simulink library "pacejka_trans"  (R2020b)
settings: Solver=ode45  StartTime=0.0  StopTime=10.0  RelTol=1e-3  EnableMultiTasking=on
undefined symbols (not defined in the file): DiscIntNeverNeededParam, par_TIR, UC_TireFy
libraries: simulink x2, $bdroot x1
(part 1 of 2)
settings Model: Creator=schultze  LastModifiedBy=ga69qig
settings DataIOCC: LimitDataPoints=on  SaveFormat=Array  SignalLoggingSaveFormat=ModelDataLogs  ReturnWorkspaceOutputs=off
settings OptimizationCC: ExpressionDepthLimit=2147483647  LifeSpan=inf
settings DebuggingCC: UnderspecifiedInitializationDetection=Classic  MergeDetectMultiDrivingBlocksExec=none  SolverPrmCheckMsg=warning  FcnCallInpInsideContextMsg=warning  AllowSymbolicDim=off  StateNameClashWarn=warning  SFUnexpectedBacktrackingDiag=warning  SFNoUnconditionalDefaultTransitionDiag=warning  SFExecutionAtInitializationDiag=none  ArithmeticOperatorsInVariantConditions=warning
settings HardwareCC: ProdBitPerPointer=32  ProdBitPerSizeT=32  ProdBitPerPtrDiffT=32  ProdLargestAtomicFloat=None  ProdIntDivRoundTo=Undefined  ProdEndianess=Unspecified  ProdWordSize=32  ProdHWDeviceType=32-bit Generic
settings ModelReferenceCC: PropagateSignalLabelsOutOfModel=off
settings SFSimCC: SimUseLocalCustomCode=off  CustomCodeUndefinedFunction=UseInterfaceOnly
settings RTWCC: RTWUseLocalCustomCode=off
settings CodeAppCC: StateflowObjectComments=on
settings GRTTargetCC: TargetLangStandard=C89/C90 (ANSI)  CombineOutputUpdateFcns=off  GRTInterface=on
settings ConfigComp: CovMetricSettings=dw  CovSaveCumulativeToWorkspaceVar=on  CovSaveSingleToWorkspaceVar=on  CovExternalEMLEnable=off

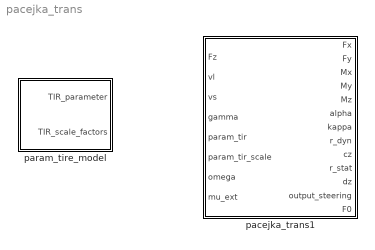
== system pacejka_trans ==
  pacejka_trans1 : Subsystem  mask{mounted_side_input=right}
      mask prompts: mounted_side_input "mounted side"
      mask init:
      | switch mounted_side_input
      |     case 1
      |         mounted_side=0;
      |     case 2
      |         mounted_side=1;
      |     case 3
      |         mounted_side=-1;
      | end
      mask TypeOptions mounted_side_input: undefined | left | right
  param_tire_model : Subsystem

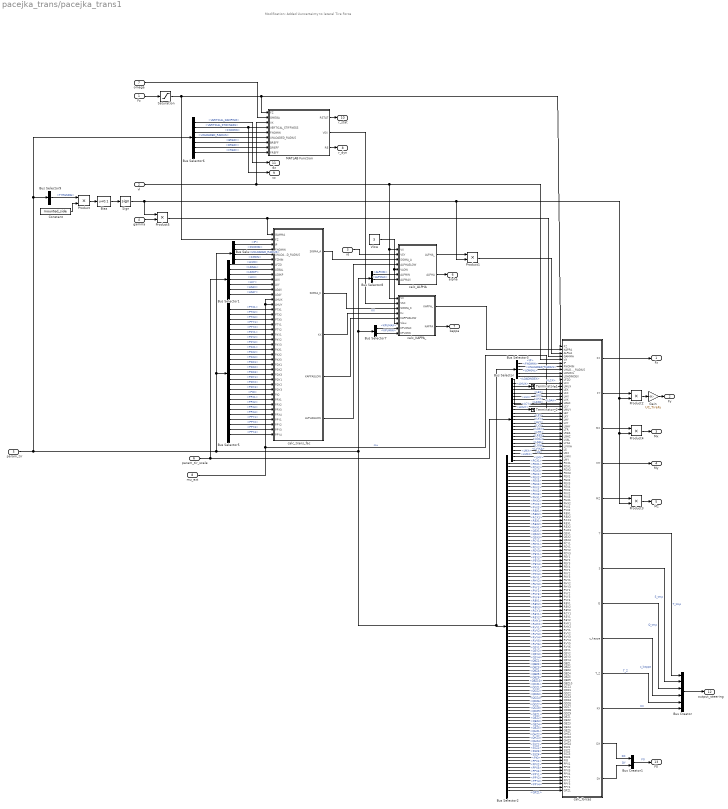
== system pacejka_trans/pacejka_trans1 ==
  note: Modification: Added Uuncertainty to lateral Tire Force
  Fz : Inport
  vl : Inport  Port=2
  vs : Inport  Port=3
  gamma : Inport  Port=4
  param_tir : Inport  Port=5
  param_tir_scale : Inport  Port=6
  omega : Inport  Port=7
  mu_ext : Inport  Port=8
  Bias : Bias  Bias=0.1
  Bus Creator : BusCreator  Inputs=6
  Bus Creator1 : BusCreator  Inputs=2
  Bus Selector : BusSelector  OutputSignals=LFZO,LCX,LMUX,LEX,LKX,LHX,LVX,LGAX,LCY,LMUY,LEY,LKY,LHY,LVY,LGAY,LTR,LRES,LGAZ,LXAL,LYKA,LVYKA,LS,LMX,LVMX,LMY
  Bus Selector1 : BusSelector  OutputSignals=LFZO,LSGAL,LSGKP,LKX,LKY,LGAX,LGAY
  Bus Selector2 : BusSelector  OutputSignals=PCX1,PDX1,PDX2,PDX3,PEX1,PEX2,PEX3,PEX4,PKX1,PKX2,PKX3,PHX1,PHX2,PVX1,PVX2,RBX1,RBX2,RCX1,REX1,REX2,RHX1,QSX1,QSX2,QSX3,PCY1,PDY1,PDY2,PDY3,PEY1,PEY2,PEY3,PEY4,PKY1,PKY2,PKY3,PHY1,PHY2,PHY3,PVY1,PVY2,PVY3,PVY4,RBY1,RBY2,RBY3,RCY1,REY1,REY2,RHY1,RHY2,RVY1,RVY2,RVY3,RVY4,RVY5,RVY6,QSY1,QSY2,QSY3,QSY4,QBZ1,QBZ2,QBZ3,QBZ4,QBZ5,QBZ9,QBZ10,QCZ1,QDZ1,QDZ2,QDZ3,QDZ4,QDZ6,QDZ7,QDZ8,QDZ9,QEZ1,QEZ2,QEZ3,QEZ4,QEZ5,QHZ1,QHZ2,QHZ3,QHZ4,SSZ1,SSZ2,SSZ3,SSZ4,PIO,PPX1,PPX2,PPX3,PPX4,PPY1,PPY2,PPY3,PPY4,QPZ1
  Bus Selector3 : BusSelector  OutputSignals=IP,FNOMIN,UNLOADED_RADIUS,LONGVL,LOADINDEX
  Bus Selector4 : BusSelector  OutputSignals=IP,FNOMIN,UNLOADED_RADIUS,FZMIN
  Bus Selector5 : BusSelector  OutputSignals=PTX1,PTX2,PTX3,PTY1,PTY2,PKY1,PKY2,PKY3,PKX1,PKX2,PKX3,PDX1,PDX2,PDX3,PDY1,PDY2,PDY3,PIO,PPX1,PPX2,PPX3,PPX4,PPY1,PPY2,PPY3,PPY4
  Bus Selector6 : BusSelector  OutputSignals=VERTICAL_DAMPING,VERTICAL_STIFFNESS,FNOMIN,UNLOADED_RADIUS,BREFF,DREFF,FREFF
  Bus Selector7 : BusSelector  OutputSignals=KPUMAX,KPUMIN
  Bus Selector8 : BusSelector  OutputSignals=ALPMIN,ALPMAX
  Bus Selector9 : BusSelector  OutputSignals=TYRESIDE
  Constant : Constant  Value=mounted_side
  Gain : Gain  Gain=UC_TireFy
  MATLAB Function : MATLAB Function  TreatAsAtomicUnit=on
  Product{,1..5} (6 alike) : Product  RndMeth=Zero
  Saturation : Saturate  UpperLimit=99999999  LowerLimit=0.001
  Sign : Signum
  Terminator_1 : Terminator
  Terminator_2 : Terminator
  Vlow : Constant  Value=3
  calc_ALPHA : Subsystem
  calc_KAPPA_ : Subsystem
  calc_forces : MATLAB Function  TreatAsAtomicUnit=on
  calc_trans_fac : MATLAB Function  TreatAsAtomicUnit=on
  Fx : Outport  VectorParamsAs1DForOutWhenUnconnected=off
  Fy : Outport  Port=2  VectorParamsAs1DForOutWhenUnconnected=off
  Mx : Outport  Port=3  VectorParamsAs1DForOutWhenUnconnected=off
  My : Outport  Port=4  VectorParamsAs1DForOutWhenUnconnected=off
  Mz : Outport  Port=5  VectorParamsAs1DForOutWhenUnconnected=off
  alpha : Outport  Port=6  VectorParamsAs1DForOutWhenUnconnected=off
  kappa : Outport  Port=7  VectorParamsAs1DForOutWhenUnconnected=off
  r_dyn : Outport  Port=8  VectorParamsAs1DForOutWhenUnconnected=off
  cz : Outport  Port=9  VectorParamsAs1DForOutWhenUnconnected=off
  r_stat : Outport  Port=10  VectorParamsAs1DForOutWhenUnconnected=off
  dz : Outport  Port=11  VectorParamsAs1DForOutWhenUnconnected=off
  output_steering : Outport  Port=12  VectorParamsAs1DForOutWhenUnconnected=off
  F0 : Outport  Port=13  VectorParamsAs1DForOutWhenUnconnected=off
  wires:
  Bus Creator1/1 -> F0/1  "F0"
  calc_forces/13(DY) -> Bus Creator1/2  "DY"
  calc_forces/12(DX) -> Bus Creator1/1  "DX"
  Bus Selector/25 -> calc_forces/35(LMY)  "<LMY>"
  calc_forces/11(KX) -> Bus Creator/6  "KX"
  Bus Selector4/1 -> calc_trans_fac/3(IP)  "<IP>"
  Bus Selector5/26 -> calc_trans_fac/41(PPY4)  "<PPY4>"
  Bus Selector5/25 -> calc_trans_fac/40(PPY3)  "<PPY3>"
  Bus Selector5/24 -> calc_trans_fac/39(PPY2)  "<PPY2>"
  Bus Selector5/23 -> calc_trans_fac/38(PPY1)  "<PPY1>"
  Bus Selector5/22 -> calc_trans_fac/37(PPX4)  "<PPX4>"
  Bus Selector5/21 -> calc_trans_fac/36(PPX3)  "<PPX3>"
  Bus Selector5/20 -> calc_trans_fac/35(PPX2)  "<PPX2>"
  Bus Selector5/19 -> calc_trans_fac/34(PPX1)  "<PPX1>"
  Bus Selector5/18 -> calc_trans_fac/33(PIO)  "<PIO>"
  Bus Selector3/1 -> calc_forces/6(IP)  "<IP>"
  Bus Selector3/5 -> calc_forces/10(LOADINDEX)  "<LOADINDEX>"
  Bus Selector3/4 -> calc_forces/9(LONGVL)  "<LONGVL>"
  Bus Selector2/99 -> calc_forces/134(QPZ1)  "<QPZ1>"
  Bus Selector2/98 -> calc_forces/133(PPY4)  "<PPY4>"
  Bus Selector2/97 -> calc_forces/132(PPY3)  "<PPY3>"
  Bus Selector2/96 -> calc_forces/131(PPY2)  "<PPY2>"
  Bus Selector2/95 -> calc_forces/130(PPY1)  "<PPY1>"
  Bus Selector2/94 -> calc_forces/129(PPX4)  "<PPX4>"
  Bus Selector2/93 -> calc_forces/128(PPX3)  "<PPX3>"
  Bus Selector2/92 -> calc_forces/127(PPX2)  "<PPX2>"
  Bus Selector2/91 -> calc_forces/126(PPX1)  "<PPX1>"
  Bus Selector2/90 -> calc_forces/125(PIO)  "<PIO>"
  calc_forces/10(T_Z) -> Bus Creator/5  "T_Z"
  calc_forces/9(c_kappa) -> Bus Creator/4  "c_kappa"
  Bus Creator/1 -> output_steering/1
  gamma/1 -> Product5/2
  calc_KAPPA_/2(KAPPA) -> kappa/1
  mu_ext/1 -> calc_forces/13(LMUX), calc_forces/20(LMUY), calc_trans_fac/15(LMUY), calc_trans_fac/14(LMUX)  "mu"
  Vlow/1 -> calc_ALPHA/5(VLOW), calc_KAPPA_/6(Vlow)
  Bus Selector1/5 -> calc_trans_fac/11(LKY)  "<LKY>"
  calc_trans_fac/5(ALPHASLOW) -> calc_ALPHA/4(ALPHASLOW)
  Bus Selector5/7 -> calc_trans_fac/22(PKY2)  "<PKY2>"
  Bus Selector5/6 -> calc_trans_fac/21(PKY1)  "<PKY1>"
  Bus Selector5/17 -> calc_trans_fac/32(PDY3)  "<PDY3>"
  Bus Selector5/16 -> calc_trans_fac/31(PDY2)  "<PDY2>"
  Bus Selector5/15 -> calc_trans_fac/30(PDY1)  "<PDY1>"
  Bus Selector1/7 -> calc_trans_fac/13(LGAY)  "<LGAY>"
  calc_trans_fac/4(KAPPASLOW) -> calc_KAPPA_/5(KAPPASLOW)
  Bus Selector5/14 -> calc_trans_fac/29(PDX3)  "<PDX3>"
  Bus Selector5/13 -> calc_trans_fac/28(PDX2)  "<PDX2>"
  Bus Selector5/12 -> calc_trans_fac/27(PDX1)  "<PDX1>"
  Bus Selector1/6 -> calc_trans_fac/12(LGAX)  "<LGAX>"
  Bus Selector5/11 -> calc_trans_fac/26(PKX3)  "<PKX3>"
  Bus Selector5/10 -> calc_trans_fac/25(PKX2)  "<PKX2>"
  Bus Selector5/9 -> calc_trans_fac/24(PKX1)  "<PKX1>"
  Bus Selector1/4 -> calc_trans_fac/10(LKX)  "<LKX>"
  calc_trans_fac/3(KX) -> calc_KAPPA_/4(Kx)  "KX"
  vl/1 -> calc_forces/5(VX), calc_ALPHA/1(VX), calc_KAPPA_/1(VX), MATLAB Function/3(VX)
  Bus Selector6/7 -> MATLAB Function/9(FREFF)  "<FREFF>"
  Bus Selector6/6 -> MATLAB Function/8(DREFF)  "<DREFF>"
  Bus Selector6/5 -> MATLAB Function/7(BREFF)  "<BREFF>"
  Bus Selector4/4 -> calc_trans_fac/6(FZMIN)  "<FZMIN>"
  calc_ALPHA/1(ALPHA_) -> Product1/1
  calc_trans_fac/1(SIGMA_A) -> calc_ALPHA/3(SIGMA_A)
  calc_trans_fac/2(SIGMA_K) -> calc_KAPPA_/3(SIGMA_K)
  vs/1 -> calc_ALPHA/2(VSY)
  Fz/1 -> Saturation/1
  Product5/1 -> calc_forces/4(GAMMA), calc_trans_fac/1(GAMMA)
  param_tir_scale/1 -> Bus Selector/1, Bus Selector1/1
  Bus Selector/1 -> calc_forces/11(LFZO)  "<LFZO>"
  Bus Selector/2 -> calc_forces/12(LCX)  "<LCX>"
  Bus Selector/4 -> calc_forces/14(LEX)  "<LEX>"
  Bus Selector/5 -> calc_forces/15(LKX)  "<LKX>"
  Bus Selector/6 -> calc_forces/16(LHX)  "<LHX>"
  Bus Selector/7 -> calc_forces/17(LVX)  "<LVX>"
  Bus Selector/8 -> calc_forces/18(LGAX)  "<LGAX>"
  Bus Selector/9 -> calc_forces/19(LCY)  "<LCY>"
  Bus Selector/11 -> calc_forces/21(LEY)  "<LEY>"
  Bus Selector/12 -> calc_forces/22(LKY)  "<LKY>"
  Bus Selector/13 -> calc_forces/23(LHY)  "<LHY>"
  Bus Selector/14 -> calc_forces/24(LVY)  "<LVY>"
  Bus Selector/15 -> calc_forces/25(LGAY)  "<LGAY>"
  Bus Selector/16 -> calc_forces/26(LTR)  "<LTR>"
  Bus Selector/17 -> calc_forces/27(LRES)  "<LRES>"
  Bus Selector/18 -> calc_forces/28(LGAZ)  "<LGAZ>"
  Bus Selector/19 -> calc_forces/29(LXAL)  "<LXAL>"
  Bus Selector/20 -> calc_forces/30(LYKA)  "<LYKA>"
  Bus Selector/21 -> calc_forces/31(LVYKA)  "<LVYKA>"
  Bus Selector/22 -> calc_forces/32(LS)  "<LS>"
  Bus Selector/23 -> calc_forces/33(LMX)  "<LMX>"
  Bus Selector/24 -> calc_forces/34(LVMX)  "<LVMX>"
  Bus Selector1/1 -> calc_trans_fac/7(LFZO)  "<LFZO>"
  Bus Selector1/2 -> calc_trans_fac/8(LSGAL)  "<LSGAL>"
  Bus Selector1/3 -> calc_trans_fac/9(LSGKP)  "<LSGKP>"
  param_tir/1 -> Bus Selector2/1, Bus Selector3/1, Bus Selector7/1, Bus Selector8/1, Bus Selector5/1, Bus Selector4/1, Bus Selector6/1, Bus Selector9/1
  Bus Selector3/2 -> calc_forces/7(FNOMIN)  "<FNOMIN>"
  Bus Selector3/3 -> calc_forces/8(UNLOADED_RADIUS)  "<UNLOADED_RADIUS>"
  Bus Selector2/1 -> calc_forces/36(PCX1)  "<PCX1>"
  Bus Selector2/2 -> calc_forces/37(PDX1)  "<PDX1>"
  Bus Selector2/3 -> calc_forces/38(PDX2)  "<PDX2>"
  Bus Selector2/4 -> calc_forces/39(PDX3)  "<PDX3>"
  Bus Selector2/5 -> calc_forces/40(PEX1)  "<PEX1>"
  Bus Selector2/6 -> calc_forces/41(PEX2)  "<PEX2>"
  Bus Selector2/7 -> calc_forces/42(PEX3)  "<PEX3>"
  Bus Selector2/8 -> calc_forces/43(PEX4)  "<PEX4>"
  Bus Selector2/9 -> calc_forces/44(PKX1)  "<PKX1>"
  Bus Selector2/10 -> calc_forces/45(PKX2)  "<PKX2>"
  Bus Selector2/11 -> calc_forces/46(PKX3)  "<PKX3>"
  Bus Selector2/12 -> calc_forces/47(PHX1)  "<PHX1>"
  Bus Selector2/13 -> calc_forces/48(PHX2)  "<PHX2>"
  Bus Selector2/14 -> calc_forces/49(PVX1)  "<PVX1>"
  Bus Selector2/15 -> calc_forces/50(PVX2)  "<PVX2>"
  Bus Selector2/16 -> calc_forces/51(RBX1)  "<RBX1>"
  Bus Selector2/17 -> calc_forces/52(RBX2)  "<RBX2>"
  Bus Selector2/18 -> calc_forces/53(RCX1)  "<RCX1>"
  Bus Selector2/19 -> calc_forces/54(REX1)  "<REX1>"
  Bus Selector2/20 -> calc_forces/55(REX2)  "<REX2>"
  Bus Selector2/21 -> calc_forces/56(RHX1)  "<RHX1>"
  Bus Selector2/22 -> calc_forces/57(QSX1)  "<QSX1>"
  Bus Selector2/23 -> calc_forces/58(QSX2)  "<QSX2>"
  Bus Selector2/24 -> calc_forces/59(QSX3)  "<QSX3>"
  Bus Selector2/25 -> calc_forces/60(PCY1)  "<PCY1>"
  Bus Selector2/26 -> calc_forces/61(PDY1)  "<PDY1>"
  Bus Selector2/27 -> calc_forces/62(PDY2)  "<PDY2>"
  Bus Selector2/28 -> calc_forces/63(PDY3)  "<PDY3>"
  Bus Selector2/29 -> calc_forces/64(PEY1)  "<PEY1>"
  Bus Selector2/30 -> calc_forces/65(PEY2)  "<PEY2>"
  Bus Selector2/31 -> calc_forces/66(PEY3)  "<PEY3>"
  Bus Selector2/32 -> calc_forces/67(PEY4)  "<PEY4>"
  Bus Selector2/33 -> calc_forces/68(PKY1)  "<PKY1>"
  Bus Selector2/34 -> calc_forces/69(PKY2)  "<PKY2>"
  Bus Selector2/35 -> calc_forces/70(PKY3)  "<PKY3>"
  Bus Selector2/36 -> calc_forces/71(PHY1)  "<PHY1>"
  Bus Selector2/37 -> calc_forces/72(PHY2)  "<PHY2>"
  Bus Selector2/38 -> calc_forces/73(PHY3)  "<PHY3>"
  Bus Selector2/39 -> calc_forces/74(PVY1)  "<PVY1>"
  Bus Selector2/40 -> calc_forces/75(PVY2)  "<PVY2>"
  Bus Selector2/41 -> calc_forces/76(PVY3)  "<PVY3>"
  Bus Selector2/42 -> calc_forces/77(PVY4)  "<PVY4>"
  Bus Selector2/43 -> calc_forces/78(RBY1)  "<RBY1>"
  Bus Selector2/44 -> calc_forces/79(RBY2)  "<RBY2>"
  Bus Selector2/45 -> calc_forces/80(RBY3)  "<RBY3>"
  Bus Selector2/46 -> calc_forces/81(RCY1)  "<RCY1>"
  Bus Selector2/47 -> calc_forces/82(REY1)  "<REY1>"
  Bus Selector2/48 -> calc_forces/83(REY2)  "<REY2>"
  Bus Selector2/49 -> calc_forces/84(RHY1)  "<RHY1>"
  Bus Selector2/50 -> calc_forces/85(RHY2)  "<RHY2>"
  Bus Selector2/51 -> calc_forces/86(RVY1)  "<RVY1>"
  Bus Selector2/52 -> calc_forces/87(RVY2)  "<RVY2>"
  Bus Selector2/53 -> calc_forces/88(RVY3)  "<RVY3>"
  Bus Selector2/54 -> calc_forces/89(RVY4)  "<RVY4>"
  Bus Selector2/55 -> calc_forces/90(RVY5)  "<RVY5>"
  Bus Selector2/56 -> calc_forces/91(RVY6)  "<RVY6>"
  Bus Selector2/57 -> calc_forces/92(QSY1)  "<QSY1>"
  Bus Selector2/58 -> calc_forces/93(QSY2)  "<QSY2>"
  Bus Selector2/59 -> calc_forces/94(QSY3)  "<QSY3>"
  Bus Selector2/60 -> calc_forces/95(QSY4)  "<QSY4>"
  Bus Selector2/61 -> calc_forces/96(QBZ1)  "<QBZ1>"
  Bus Selector2/62 -> calc_forces/97(QBZ2)  "<QBZ2>"
  Bus Selector2/63 -> calc_forces/98(QBZ3)  "<QBZ3>"
  Bus Selector2/64 -> calc_forces/99(QBZ4)  "<QBZ4>"
  Bus Selector2/65 -> calc_forces/100(QBZ5)  "<QBZ5>"
  Bus Selector2/66 -> calc_forces/101(QBZ9)  "<QBZ9>"
  Bus Selector2/67 -> calc_forces/102(QBZ10)  "<QBZ10>"
  Bus Selector2/68 -> calc_forces/103(QCZ1)  "<QCZ1>"
  Bus Selector2/69 -> calc_forces/104(QDZ1)  "<QDZ1>"
  Bus Selector2/70 -> calc_forces/105(QDZ2)  "<QDZ2>"
  Bus Selector2/71 -> calc_forces/106(QDZ3)  "<QDZ3>"
  Bus Selector2/72 -> calc_forces/107(QDZ4)  "<QDZ4>"
  Bus Selector2/73 -> calc_forces/108(QDZ6)  "<QDZ6>"
  Bus Selector2/74 -> calc_forces/109(QDZ7)  "<QDZ7>"
  Bus Selector2/75 -> calc_forces/110(QDZ8)  "<QDZ8>"
  Bus Selector2/76 -> calc_forces/111(QDZ9)  "<QDZ9>"
  Bus Selector2/77 -> calc_forces/112(QEZ1)  "<QEZ1>"
  Bus Selector2/78 -> calc_forces/113(QEZ2)  "<QEZ2>"
  Bus Selector2/79 -> calc_forces/114(QEZ3)  "<QEZ3>"
  Bus Selector2/80 -> calc_forces/115(QEZ4)  "<QEZ4>"
  Bus Selector2/81 -> calc_forces/116(QEZ5)  "<QEZ5>"
  Bus Selector2/82 -> calc_forces/117(QHZ1)  "<QHZ1>"
  Bus Selector2/83 -> calc_forces/118(QHZ2)  "<QHZ2>"
  Bus Selector2/84 -> calc_forces/119(QHZ3)  "<QHZ3>"
  Bus Selector2/85 -> calc_forces/120(QHZ4)  "<QHZ4>"
  Bus Selector2/86 -> calc_forces/121(SSZ1)  "<SSZ1>"
  Bus Selector2/87 -> calc_forces/122(SSZ2)  "<SSZ2>"
  Bus Selector2/88 -> calc_forces/123(SSZ3)  "<SSZ3>"
  Bus Selector2/89 -> calc_forces/124(SSZ4)  "<SSZ4>"
  Bus Selector5/1 -> calc_trans_fac/16(PTX1)  "<PTX1>"
  Bus Selector5/2 -> calc_trans_fac/17(PTX2)  "<PTX2>"
  Bus Selector5/3 -> calc_trans_fac/18(PTX3)  "<PTX3>"
  Bus Selector5/4 -> calc_trans_fac/19(PTY1)  "<PTY1>"
  Bus Selector5/5 -> calc_trans_fac/20(PTY2)  "<PTY2>"
  Bus Selector5/8 -> calc_trans_fac/23(PKY3)  "<PKY3>"
  Bus Selector4/2 -> calc_trans_fac/4(FNOMIN)  "<FNOMIN>"
  Bus Selector4/3 -> calc_trans_fac/5(UNLOADED_RADIUS)  "<UNLOADED_RADIUS>"
  MATLAB Function/2(VSX) -> calc_KAPPA_/2(VSX)
  Bus Selector6/2 -> MATLAB Function/4(VERTICAL_STIFFNESS), cz/1  "<VERTICAL_STIFFNESS>"
  Bus Selector6/3 -> MATLAB Function/5(FNOMIN)  "<FNOMIN>"
  Bus Selector6/4 -> MATLAB Function/6(UNLOADED_RADIUS)  "<UNLOADED_RADIUS>"
  omega/1 -> MATLAB Function/2(OMEGA)
  MATLAB Function/3(RE) -> r_dyn/1
  calc_forces/4(MY) -> My/1
  calc_forces/1(FX) -> Fx/1
  Bus Selector/10 -> Terminator_2/1  "<LMUY>"
  Bus Selector7/1 -> calc_KAPPA_/7(KPUMAX)  "<KPUMAX>"
  Bus Selector7/2 -> calc_KAPPA_/8(KPUMIN)  "<KPUMIN>"
  Bus Selector8/1 -> calc_ALPHA/6(ALPMIN)  "<ALPMIN>"
  Bus Selector8/2 -> calc_ALPHA/7(ALPMAX)  "<ALPMAX>"
  Product1/1 -> calc_forces/3(ALPHA)
  Bus Selector/3 -> Terminator_1/1  "<LMUX>"
  Bus Selector9/1 -> Product/1  "<TYRESIDE>"
  Constant/1 -> Product/2
  Product/1 -> Bias/1
  Bias/1 -> Sign/1
  Sign/1 -> Product1/2, Product3/2, Product4/2, Product2/2, Product5/1
  Product2/1 -> Gain/1
  Product3/1 -> Mz/1
  calc_forces/5(MZ) -> Product3/1
  Product4/1 -> Mx/1
  calc_forces/3(MX) -> Product4/1
  MATLAB Function/1(RSTAT) -> r_stat/1
  Bus Selector6/1 -> dz/1  "<VERTICAL_DAMPING>"
  Saturation/1 -> calc_forces/1(FZ), MATLAB Function/1(FZ), calc_trans_fac/2(FZ)
  calc_forces/2(FY) -> Product2/1
  calc_ALPHA/2(ALPHA) -> alpha/1
  calc_forces/6(T) -> Bus Creator/1  "T_tmp"
  calc_forces/7(S) -> Bus Creator/2  "S_tmp"
  calc_forces/8(Q) -> Bus Creator/3  "Q_tmp"
  calc_KAPPA_/1(KAPPA_) -> calc_forces/2(KAPPA)
  Gain/1 -> Fy/1

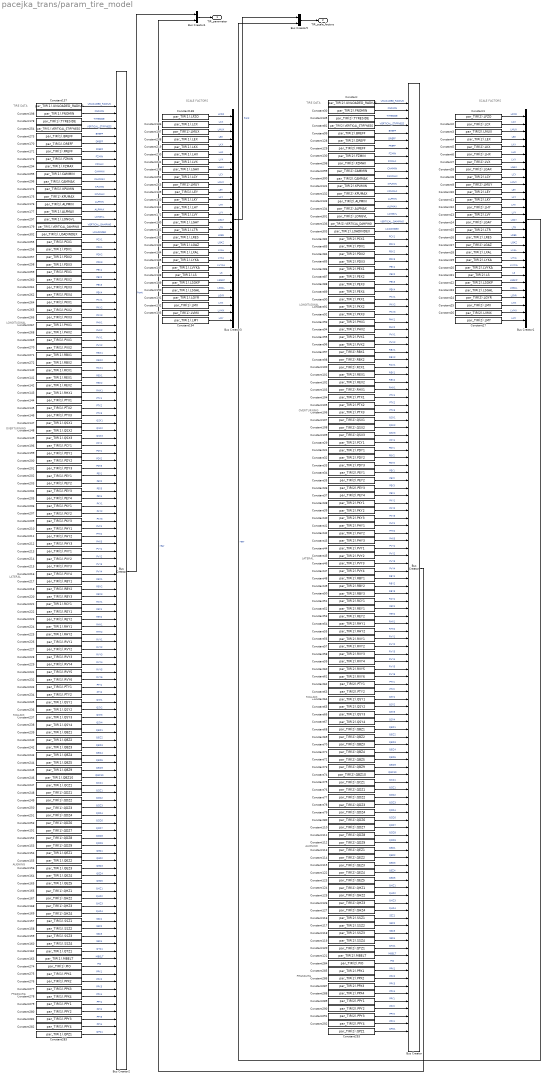
== system pacejka_trans/param_tire_model ==
  note: SCALE FACTORS
  note: TIRE DATA
  note: LONGITUDINAL
  note: LATERAL
  note: OVERTURNING
  note: ROLLING
  note: ALIGNING
  note: SCALE FACTORS
  note: TIRE DATA
  note: LONGITUDINAL
  note: LATERAL
  note: OVERTURNING
  note: ROLLING
  note: ALIGNING
  note: PRESSURE
  note: PRESSURE
  Bus Creator : BusCreator  Inputs=124
  Bus Creator1 : BusCreator  Inputs=28
  Bus Creator2 : BusCreator  Inputs=124
  Bus Creator3 : BusCreator  Inputs=28
  Bus Creator4 : BusCreator  Inputs=2
  Bus Creator5 : BusCreator  Inputs=2
  Constant : Constant  Value=par_TIR(2).UNLOADED_RADIUS
  Constant1 : Constant  Value=par_TIR(2).LFZO
  Constant10 : Constant  Value=par_TIR(2).LEY
  Constant100 : Constant  Value=par_TIR(2).RCX1
  Constant101 : Constant  Value=par_TIR(2).REX1
  Constant102 : Constant  Value=par_TIR(2).REX2
  Constant103 : Constant  Value=par_TIR(2).RHX1
  Constant104 : Constant  Value=par_TIR(2).PTX1
  Constant105 : Constant  Value=par_TIR(2).PTX2
  Constant106 : Constant  Value=par_TIR(2).PTX3
  Constant107 : Constant  Value=par_TIR(2).QSX1
  Constant108 : Constant  Value=par_TIR(2).QSX2
  Constant109 : Constant  Value=par_TIR(2).QSX3
  Constant11 : Constant  Value=par_TIR(2).LKY
  Constant110 : Constant  Value=par_TIR(2).QDZ7
  Constant111 : Constant  Value=par_TIR(2).QDZ8
  Constant112 : Constant  Value=par_TIR(2).QDZ9
  Constant113 : Constant  Value=par_TIR(2).QEZ1
  Constant114 : Constant  Value=par_TIR(2).QEZ2
  Constant115 : Constant  Value=par_TIR(2).QEZ3
  Constant116 : Constant  Value=par_TIR(2).SSZ1
  Constant117 : Constant  Value=par_TIR(2).SSZ2
  Constant118 : Constant  Value=par_TIR(2).SSZ3
  Constant119 : Constant  Value=par_TIR(2).SSZ4
  Constant12 : Constant  Value=par_TIR(2).LHY
  Constant120 : Constant  Value=par_TIR(2).QTZ1
  Constant121 : Constant  Value=par_TIR(2).MBELT
  Constant122 : Constant  Value=par_TIR(2).QEZ4
  Constant123 : Constant  Value=par_TIR(2).QEZ5
  Constant124 : Constant  Value=par_TIR(2).QHZ1
  Constant125 : Constant  Value=par_TIR(2).QHZ2
  Constant126 : Constant  Value=par_TIR(2).QHZ3
  Constant127 : Constant  Value=par_TIR(2).QHZ4
  Constant128 : Constant  Value=par_TIR(2).DREFF
  Constant129 : Constant  Value=par_TIR(2).FREFF
  Constant13 : Constant  Value=par_TIR(2).LVY
  Constant130 : Constant  Value=par_TIR(2).FZMIN
  Constant131 : Constant  Value=par_TIR(2).KPUMIN
  Constant132 : Constant  Value=par_TIR(2).KPUMAX
  Constant133 : Constant  Value=par_TIR(2).ALPMIN
  Constant134 : Constant  Value=par_TIR(2).ALPMAX
  Constant135 : Constant  Value=par_TIR(2).TYRESIDE
  Constant136 : Constant  Value=par_TIR(2).VERTICAL_DAMPING
  Constant137 : Constant  Value=par_TIR(1).UNLOADED_RADIUS
  Constant138 : Constant  Value=par_TIR(1).LFZO
  Constant139 : Constant  Value=par_TIR(1).LEY
  Constant14 : Constant  Value=par_TIR(2).LGAY
  Constant140 : Constant  Value=par_TIR(1).RCX1
  Constant141 : Constant  Value=par_TIR(1).REX1
  Constant142 : Constant  Value=par_TIR(1).REX2
  Constant143 : Constant  Value=par_TIR(1).RHX1
  Constant144 : Constant  Value=par_TIR(1).PTX1
  Constant145 : Constant  Value=par_TIR(1).PTX2
  Constant146 : Constant  Value=par_TIR(1).PTX3
  Constant147 : Constant  Value=par_TIR(1).QSX1
  Constant148 : Constant  Value=par_TIR(1).QSX2
  Constant149 : Constant  Value=par_TIR(1).QSX3
  Constant15 : Constant  Value=par_TIR(2).LTR
  Constant150 : Constant  Value=par_TIR(1).LKY
  Constant151 : Constant  Value=par_TIR(1).QDZ7
  Constant152 : Constant  Value=par_TIR(1).QDZ8
  Constant153 : Constant  Value=par_TIR(1).QDZ9
  Constant154 : Constant  Value=par_TIR(1).QEZ1
  Constant155 : Constant  Value=par_TIR(1).QEZ2
  Constant156 : Constant  Value=par_TIR(1).QEZ3
  Constant157 : Constant  Value=par_TIR(1).SSZ1
  Constant158 : Constant  Value=par_TIR(1).SSZ2
  Constant159 : Constant  Value=par_TIR(1).SSZ3
  Constant16 : Constant  Value=par_TIR(2).LRES
  Constant160 : Constant  Value=par_TIR(1).SSZ4
  Constant161 : Constant  Value=par_TIR(1).LHY
  Constant162 : Constant  Value=par_TIR(1).QTZ1
  Constant163 : Constant  Value=par_TIR(1).MBELT
  Constant164 : Constant  Value=par_TIR(1).QEZ4
  Constant165 : Constant  Value=par_TIR(1).QEZ5
  Constant166 : Constant  Value=par_TIR(1).QHZ1
  Constant167 : Constant  Value=par_TIR(1).QHZ2
  Constant168 : Constant  Value=par_TIR(1).QHZ3
  Constant169 : Constant  Value=par_TIR(1).QHZ4
  Constant17 : Constant  Value=par_TIR(2).LGAZ
  Constant170 : Constant  Value=par_TIR(1).DREFF
  Constant171 : Constant  Value=par_TIR(1).FREFF
  Constant172 : Constant  Value=par_TIR(1).LVY
  Constant173 : Constant  Value=par_TIR(1).FZMIN
  Constant174 : Constant  Value=par_TIR(1).KPUMIN
  Constant175 : Constant  Value=par_TIR(1).KPUMAX
  Constant176 : Constant  Value=par_TIR(1).ALPMIN
  Constant177 : Constant  Value=par_TIR(1).ALPMAX
  Constant178 : Constant  Value=par_TIR(1).TYRESIDE
  Constant179 : Constant  Value=par_TIR(1).VERTICAL_DAMPING
  Constant18 : Constant  Value=par_TIR(2).LXAL
  Constant180 : Constant  Value=par_TIR(1).LGAY
  Constant181 : Constant  Value=par_TIR(1).LTR
  Constant182 : Constant  Value=par_TIR(1).LRES
  Constant183 : Constant  Value=par_TIR(1).LGAZ
  Constant184 : Constant  Value=par_TIR(1).LXAL
  Constant185 : Constant  Value=par_TIR(1).LYKA
  Constant186 : Constant  Value=par_TIR(1).LCX
  Constant187 : Constant  Value=par_TIR(1).LVYKA
  Constant188 : Constant  Value=par_TIR(1).LS
  Constant189 : Constant  Value=par_TIR(1).LSGKP
  Constant19 : Constant  Value=par_TIR(2).LYKA
  Constant190 : Constant  Value=par_TIR(1).LSGAL
  Constant191 : Constant  Value=par_TIR(1).LGYR
  Constant192 : Constant  Value=par_TIR(1).LMX
  Constant193 : Constant  Value=par_TIR(1).LVMX
  Constant194 : Constant  Value=par_TIR(1).LMY
  Constant195 : Constant  Value=par_TIR(1).LGAX
  Constant196 : Constant  Value=par_TIR(1).PCY1
  Constant197 : Constant  Value=par_TIR(1).LMUX
  Constant198 : Constant  Value=par_TIR(1).FNOMIN
  Constant199 : Constant  Value=par_TIR(1).PDY1
  Constant2 : Constant  Value=par_TIR(2).LCX
  Constant20 : Constant  Value=par_TIR(2).LVYKA
  Constant200 : Constant  Value=par_TIR(1).PDY2
  Constant201 : Constant  Value=par_TIR(1).PDY3
  Constant202 : Constant  Value=par_TIR(1).PEY1
  Constant203 : Constant  Value=par_TIR(1).PEY2
  Constant204 : Constant  Value=par_TIR(1).PEY3
  Constant205 : Constant  Value=par_TIR(1).PEY4
  Constant206 : Constant  Value=par_TIR(1).PKY1
  Constant207 : Constant  Value=par_TIR(1).PKY2
  Constant208 : Constant  Value=par_TIR(1).LEX
  Constant209 : Constant  Value=par_TIR(1).PKY3
  Constant21 : Constant  Value=par_TIR(2).LS
  Constant210 : Constant  Value=par_TIR(1).PHY1
  Constant211 : Constant  Value=par_TIR(1).PHY2
  Constant212 : Constant  Value=par_TIR(1).PHY3
  Constant213 : Constant  Value=par_TIR(1).PVY1
  Constant214 : Constant  Value=par_TIR(1).PVY2
  Constant215 : Constant  Value=par_TIR(1).PVY3
  Constant216 : Constant  Value=par_TIR(1).PVY4
  Constant217 : Constant  Value=par_TIR(1).RBY1
  Constant218 : Constant  Value=par_TIR(1).RBY2
  Constant219 : Constant  Value=par_TIR(1).LKX
  Constant22 : Constant  Value=par_TIR(2).LSGKP
  Constant220 : Constant  Value=par_TIR(1).RBY3
  Constant221 : Constant  Value=par_TIR(1).RCY1
  Constant222 : Constant  Value=par_TIR(1).REY1
  Constant223 : Constant  Value=par_TIR(1).REY2
  Constant224 : Constant  Value=par_TIR(1).RHY1
  Constant225 : Constant  Value=par_TIR(1).RHY2
  Constant226 : Constant  Value=par_TIR(1).RVY1
  Constant227 : Constant  Value=par_TIR(1).RVY2
  Constant228 : Constant  Value=par_TIR(1).RVY3
  Constant229 : Constant  Value=par_TIR(1).RVY4
  Constant23 : Constant  Value=par_TIR(2).LSGAL
  Constant230 : Constant  Value=par_TIR(1).LHX
  Constant231 : Constant  Value=par_TIR(1).RVY5
  Constant232 : Constant  Value=par_TIR(1).RVY6
  Constant233 : Constant  Value=par_TIR(1).PTY1
  Constant234 : Constant  Value=par_TIR(1).PTY2
  Constant235 : Constant  Value=par_TIR(1).QSY1
  Constant236 : Constant  Value=par_TIR(1).QSY2
  Constant237 : Constant  Value=par_TIR(1).QSY3
  Constant238 : Constant  Value=par_TIR(1).QSY4
  Constant239 : Constant  Value=par_TIR(1).QBZ1
  Constant24 : Constant  Value=par_TIR(2).LGYR
  Constant240 : Constant  Value=par_TIR(1).QBZ2
  Constant241 : Constant  Value=par_TIR(1).LVX
  Constant242 : Constant  Value=par_TIR(1).QBZ3
  Constant243 : Constant  Value=par_TIR(1).QBZ4
  Constant244 : Constant  Value=par_TIR(1).QBZ5
  Constant245 : Constant  Value=par_TIR(1).QBZ9
  Constant246 : Constant  Value=par_TIR(1).QBZ10
  Constant247 : Constant  Value=par_TIR(1).QCZ1
  Constant248 : Constant  Value=par_TIR(1).QDZ1
  Constant249 : Constant  Value=par_TIR(1).QDZ2
  Constant25 : Constant  Value=par_TIR(2).LMX
  Constant250 : Constant  Value=par_TIR(1).QDZ3
  Constant251 : Constant  Value=par_TIR(1).QDZ4
  Constant252 : Constant  Value=par_TIR(1).LCY
  Constant253 : Constant  Value=par_TIR(1).QDZ6
  Constant254 : Constant  Value=par_TIR(1).VERTICAL_STIFFNESS
  Constant255 : Constant  Value=par_TIR(1).PCX1
  Constant256 : Constant  Value=par_TIR(1).PDX1
  Constant257 : Constant  Value=par_TIR(1).PDX2
  Constant258 : Constant  Value=par_TIR(1).PDX3
  Constant259 : Constant  Value=par_TIR(1).PEX1
  Constant26 : Constant  Value=par_TIR(2).LVMX
  Constant260 : Constant  Value=par_TIR(1).PEX2
  Constant261 : Constant  Value=par_TIR(1).PEX3
  Constant262 : Constant  Value=par_TIR(1).PEX4
  Constant263 : Constant  Value=par_TIR(1).LMUY
  Constant264 : Constant  Value=par_TIR(1).PKX1
  Constant265 : Constant  Value=par_TIR(1).PKX2
  Constant266 : Constant  Value=par_TIR(1).PKX3
  Constant267 : Constant  Value=par_TIR(1).PHX1
  Constant268 : Constant  Value=par_TIR(1).PHX2
  Constant269 : Constant  Value=par_TIR(1).PVX1
  Constant27 : Constant  Value=par_TIR(2).LMY
  Constant270 : Constant  Value=par_TIR(1).PVX2
  Constant271 : Constant  Value=par_TIR(1).RBX1
  Constant272 : Constant  Value=par_TIR(1).RBX2
  Constant273 : Constant  Value=par_TIR(1).BREFF
  Constant274 : Constant  RequirementInfo="{}  %GIDa_26266586_498b_462f_b489_3d0c6574960f"  Value=par_TIR(1).PIO
  Constant275 : Constant  RequirementInfo={} %GIDa_bd3446b4_e75b_42cc_93fc_63d702bdba05  Value=par_TIR(1).PPX1
  Constant276 : Constant  RequirementInfo={} %GIDa_e7183a53_319d_4b2a_a098_83896b26e061  Value=par_TIR(1).PPX2
  Constant277 : Constant  RequirementInfo={} %GIDa_4d8b6861_cb82_4b47_965b_978958cda42f  Value=par_TIR(1).PPX3
  Constant278 : Constant  RequirementInfo={} %GIDa_c0a2bdc4_fdde_4852_836d_5878f0e5080b  Value=par_TIR(1).PPX4
  Constant279 : Constant  RequirementInfo={} %GIDa_259e4558_aa3a_40ca_8d3a_68c9cc3aff06  Value=par_TIR(1).PPY1
  Constant28 : Constant  Value=par_TIR(2).LGAX
  Constant280 : Constant  RequirementInfo={} %GIDa_19e9e64b_4c09_4622_8f00_2f4be9e7e16b  Value=par_TIR(1).PPY2
  Constant281 : Constant  RequirementInfo={} %GIDa_9a02291b_2d1e_49a5_a1e4_b19d87d3265f  Value=par_TIR(1).PPY3
  Constant282 : Constant  RequirementInfo={} %GIDa_ecd77677_9c33_4f16_bf1f_0a0632ce1b6d  Value=par_TIR(1).PPY4
  Constant283 : Constant  RequirementInfo={} %GIDa_3542e054_4fbb_4233_8b5e_2c203789807f  Value=par_TIR(1).QPZ1
  Constant284 : Constant  RequirementInfo={} %GIDa_a6cea8bb_6b90_497f_8a27_172ddd318988  Value=par_TIR(2).PIO
  Constant285 : Constant  RequirementInfo={} %GIDa_869ee301_e46e_4e3e_98d5_441bb0b60ee2  Value=par_TIR(2).PPX1
  Constant286 : Constant  RequirementInfo={} %GIDa_2fa7aad5_0b6f_4270_a9fc_fef63194a323  Value=par_TIR(2).PPX2
  Constant287 : Constant  RequirementInfo={} %GIDa_7722773f_46a5_4b48_9921_1b7dc0ffce5d  Value=par_TIR(2).PPX3
  Constant288 : Constant  RequirementInfo={} %GIDa_9b3370dd_7ca6_42c6_ae76_155bd0b3f77a  Value=par_TIR(2).PPX4
  Constant289 : Constant  RequirementInfo={} %GIDa_ebf4fb2f_cc6e_4f60_8b6d_1fa2dededda2  Value=par_TIR(2).PPY1
  Constant29 : Constant  Value=par_TIR(2).PCY1
  Constant290 : Constant  RequirementInfo={} %GIDa_46454242_b81e_41e5_9fcb_0940f6cc9231  Value=par_TIR(2).PPY2
  Constant291 : Constant  RequirementInfo={} %GIDa_9261926a_8ebc_4edf_afdf_1d43d1bd8012  Value=par_TIR(2).PPY3
  Constant292 : Constant  RequirementInfo={} %GIDa_37a6ca2e_28ac_4e3d_851e_41ea970db34f  Value=par_TIR(2).PPY4
  Constant293 : Constant  RequirementInfo={} %GIDa_06c45289_4ba3_4f48_9048_3ee6adfd56e1  Value=par_TIR(2).QPZ1
  Constant294 : Constant  Value=par_TIR(1).FZMAX
  Constant295 : Constant  Value=par_TIR(1).CAMMIN
  Constant296 : Constant  Value=par_TIR(1).CAMMAX
  Constant297 : Constant  Value=par_TIR(1).LONGVL
  Constant298 : Constant  Value=par_TIR(2).FZMAX
  Constant299 : Constant  Value=par_TIR(2).CAMMIN
  Constant3 : Constant  Value=par_TIR(2).LMUX
  Constant30 : Constant  Value=par_TIR(2).FNOMIN
  Constant300 : Constant  Value=par_TIR(2).CAMMAX
  Constant301 : Constant  Value=par_TIR(2).LONGVL
  Constant302 : Constant  Value=par_TIR(1).LOADINDEX
  Constant303 : Constant  Value=par_TIR(2).LOADINDEX
  Constant31 : Constant  Value=par_TIR(2).PDY1
  Constant32 : Constant  Value=par_TIR(2).PDY2
  Constant33 : Constant  Value=par_TIR(2).PDY3
  Constant34 : Constant  Value=par_TIR(2).PEY1
  Constant35 : Constant  Value=par_TIR(2).PEY2
  Constant36 : Constant  Value=par_TIR(2).PEY3
  Constant37 : Constant  Value=par_TIR(2).PEY4
  Constant38 : Constant  Value=par_TIR(2).PKY1
  Constant39 : Constant  Value=par_TIR(2).PKY2
  Constant4 : Constant  Value=par_TIR(2).LEX
  Constant40 : Constant  Value=par_TIR(2).PKY3
  Constant41 : Constant  Value=par_TIR(2).PHY1
  Constant42 : Constant  Value=par_TIR(2).PHY2
  Constant43 : Constant  Value=par_TIR(2).PHY3
  Constant44 : Constant  Value=par_TIR(2).PVY1
  Constant45 : Constant  Value=par_TIR(2).PVY2
  Constant46 : Constant  Value=par_TIR(2).PVY3
  Constant47 : Constant  Value=par_TIR(2).PVY4
  Constant48 : Constant  Value=par_TIR(2).RBY1
  Constant49 : Constant  Value=par_TIR(2).RBY2
  Constant5 : Constant  Value=par_TIR(2).LKX
  Constant50 : Constant  Value=par_TIR(2).RBY3
  Constant51 : Constant  Value=par_TIR(2).RCY1
  Constant52 : Constant  Value=par_TIR(2).REY1
  Constant53 : Constant  Value=par_TIR(2).REY2
  Constant54 : Constant  Value=par_TIR(2).RHY1
  Constant55 : Constant  Value=par_TIR(2).RHY2
  Constant56 : Constant  Value=par_TIR(2).RVY1
  Constant57 : Constant  Value=par_TIR(2).RVY2
  Constant58 : Constant  Value=par_TIR(2).RVY3
  Constant59 : Constant  Value=par_TIR(2).RVY4
  Constant6 : Constant  Value=par_TIR(2).LHX
  Constant60 : Constant  Value=par_TIR(2).RVY5
  Constant61 : Constant  Value=par_TIR(2).RVY6
  Constant62 : Constant  Value=par_TIR(2).PTY1
  Constant63 : Constant  Value=par_TIR(2).PTY2
  Constant64 : Constant  Value=par_TIR(2).QSY1
  Constant65 : Constant  Value=par_TIR(2).QSY2
  Constant66 : Constant  Value=par_TIR(2).QSY3
  Constant67 : Constant  Value=par_TIR(2).QSY4
  Constant68 : Constant  Value=par_TIR(2).QBZ1
  Constant69 : Constant  Value=par_TIR(2).QBZ2
  Constant7 : Constant  Value=par_TIR(2).LVX
  Constant70 : Constant  Value=par_TIR(2).QBZ3
  Constant71 : Constant  Value=par_TIR(2).QBZ4
  Constant72 : Constant  Value=par_TIR(2).QBZ5
  Constant73 : Constant  Value=par_TIR(2).QBZ9
  Constant74 : Constant  Value=par_TIR(2).QBZ10
  Constant75 : Constant  Value=par_TIR(2).QCZ1
  Constant76 : Constant  Value=par_TIR(2).QDZ1
  Constant77 : Constant  Value=par_TIR(2).QDZ2
  Constant78 : Constant  Value=par_TIR(2).QDZ3
  Constant79 : Constant  Value=par_TIR(2).QDZ4
  Constant8 : Constant  Value=par_TIR(2).LCY
  Constant80 : Constant  Value=par_TIR(2).QDZ6
  Constant81 : Constant  Value=par_TIR(2).VERTICAL_STIFFNESS
  Constant82 : Constant  Value=par_TIR(2).PCX1
  Constant83 : Constant  Value=par_TIR(2).PDX1
  Constant84 : Constant  Value=par_TIR(2).PDX2
  Constant85 : Constant  Value=par_TIR(2).PDX3
  Constant86 : Constant  Value=par_TIR(2).PEX1
  Constant87 : Constant  Value=par_TIR(2).PEX2
  Constant88 : Constant  Value=par_TIR(2).PEX3
  Constant89 : Constant  Value=par_TIR(2).PEX4
  Constant9 : Constant  Value=par_TIR(2).LMUY
  Constant90 : Constant  Value=par_TIR(2).PKX1
  Constant91 : Constant  Value=par_TIR(2).PKX2
  Constant92 : Constant  Value=par_TIR(2).PKX3
  Constant93 : Constant  Value=par_TIR(2).PHX1
  Constant94 : Constant  Value=par_TIR(2).PHX2
  Constant95 : Constant  Value=par_TIR(2).PVX1
  Constant96 : Constant  Value=par_TIR(2).PVX2
  Constant97 : Constant  Value=par_TIR(2).RBX1
  Constant98 : Constant  Value=par_TIR(2).RBX2
  Constant99 : Constant  Value=par_TIR(2).BREFF
  TIR_parameter : Outport  VectorParamsAs1DForOutWhenUnconnected=off
  TIR_scale_factors : Outport  Port=2  VectorParamsAs1DForOutWhenUnconnected=off
  wires:
  Bus Creator5/1 -> TIR_scale_factors/1
  Bus Creator3/1 -> Bus Creator5/1  "front"
  Bus Creator4/1 -> TIR_parameter/1
  Bus Creator2/1 -> Bus Creator4/1  "front"
  Constant129/1 -> Bus Creator/7  "FREFF"
  Constant128/1 -> Bus Creator/6  "DREFF"
  Constant99/1 -> Bus Creator/5  "BREFF"
  Constant1/1 -> Bus Creator1/1  "LFZO"
  Constant2/1 -> Bus Creator1/2  "LCX"
  Constant3/1 -> Bus Creator1/3  "LMUX"
  Constant4/1 -> Bus Creator1/4  "LEX"
  Constant5/1 -> Bus Creator1/5  "LKX"
  Constant6/1 -> Bus Creator1/6  "LHX"
  Constant7/1 -> Bus Creator1/7  "LVX"
  Constant28/1 -> Bus Creator1/8  "LGAX"
  Constant8/1 -> Bus Creator1/9  "LCY"
  Constant9/1 -> Bus Creator1/10  "LMUY"
  Constant10/1 -> Bus Creator1/11  "LEY"
  Constant11/1 -> Bus Creator1/12  "LKY"
  Constant12/1 -> Bus Creator1/13  "LHY"
  Constant13/1 -> Bus Creator1/14  "LVY"
  Constant14/1 -> Bus Creator1/15  "LGAY"
  Constant15/1 -> Bus Creator1/16  "LTR"
  Constant16/1 -> Bus Creator1/17  "LRES"
  Constant17/1 -> Bus Creator1/18  "LGAZ"
  Constant18/1 -> Bus Creator1/19  "LXAL"
  Constant19/1 -> Bus Creator1/20  "LYKA"
  Constant20/1 -> Bus Creator1/21  "LVYKA"
  Constant21/1 -> Bus Creator1/22  "LS"
  Constant22/1 -> Bus Creator1/23  "LSGKP"
  Constant23/1 -> Bus Creator1/24  "LSGAL"
  Constant24/1 -> Bus Creator1/25  "LGYR"
  Constant25/1 -> Bus Creator1/26  "LMX"
  Constant26/1 -> Bus Creator1/27  "LVMX"
  Constant27/1 -> Bus Creator1/28  "LMY"
  Bus Creator1/1 -> Bus Creator5/2  "rear"
  Bus Creator/1 -> Bus Creator4/2  "rear"
  Constant/1 -> Bus Creator/1  "UNLOADED_RADIUS"
  Constant30/1 -> Bus Creator/2  "FNOMIN"
  Constant82/1 -> Bus Creator/19  "PCX1"
  Constant83/1 -> Bus Creator/20  "PDX1"
  Constant84/1 -> Bus Creator/21  "PDX2"
  Constant85/1 -> Bus Creator/22  "PDX3"
  Constant86/1 -> Bus Creator/23  "PEX1"
  Constant87/1 -> Bus Creator/24  "PEX2"
  Constant88/1 -> Bus Creator/25  "PEX3"
  Constant89/1 -> Bus Creator/26  "PEX4"
  Constant90/1 -> Bus Creator/27  "PKX1"
  Constant91/1 -> Bus Creator/28  "PKX2"
  Constant92/1 -> Bus Creator/29  "PKX3"
  Constant93/1 -> Bus Creator/30  "PHX1"
  Constant94/1 -> Bus Creator/31  "PHX2"
  Constant95/1 -> Bus Creator/32  "PVX1"
  Constant96/1 -> Bus Creator/33  "PVX2"
  Constant97/1 -> Bus Creator/34  "RBX1"
  Constant98/1 -> Bus Creator/35  "RBX2"
  Constant100/1 -> Bus Creator/36  "RCX1"
  Constant101/1 -> Bus Creator/37  "REX1"
  Constant102/1 -> Bus Creator/38  "REX2"
  Constant103/1 -> Bus Creator/39  "RHX1"
  Constant104/1 -> Bus Creator/40  "PTX1"
  Constant105/1 -> Bus Creator/41  "PTX2"
  Constant106/1 -> Bus Creator/42  "PTX3"
  Constant107/1 -> Bus Creator/43  "QSX1"
  Constant108/1 -> Bus Creator/44  "QSX2"
  Constant109/1 -> Bus Creator/45  "QSX3"
  Constant29/1 -> Bus Creator/46  "PCY1"
  Constant31/1 -> Bus Creator/47  "PDY1"
  Constant32/1 -> Bus Creator/48  "PDY2"
  Constant33/1 -> Bus Creator/49  "PDY3"
  Constant34/1 -> Bus Creator/50  "PEY1"
  Constant35/1 -> Bus Creator/51  "PEY2"
  Constant36/1 -> Bus Creator/52  "PEY3"
  Constant37/1 -> Bus Creator/53  "PEY4"
  Constant38/1 -> Bus Creator/54  "PKY1"
  Constant39/1 -> Bus Creator/55  "PKY2"
  Constant40/1 -> Bus Creator/56  "PKY3"
  Constant41/1 -> Bus Creator/57  "PHY1"
  Constant42/1 -> Bus Creator/58  "PHY2"
  Constant43/1 -> Bus Creator/59  "PHY3"
  Constant44/1 -> Bus Creator/60  "PVY1"
  Constant45/1 -> Bus Creator/61  "PVY2"
  Constant46/1 -> Bus Creator/62  "PVY3"
  Constant47/1 -> Bus Creator/63  "PVY4"
  Constant48/1 -> Bus Creator/64  "RBY1"
  Constant49/1 -> Bus Creator/65  "RBY2"
  Constant50/1 -> Bus Creator/66  "RBY3"
  Constant51/1 -> Bus Creator/67  "RCY1"
  Constant52/1 -> Bus Creator/68  "REY1"
  Constant53/1 -> Bus Creator/69  "REY2"
  Constant54/1 -> Bus Creator/70  "RHY1"
  Constant55/1 -> Bus Creator/71  "RHY2"
  Constant56/1 -> Bus Creator/72  "RVY1"
  Constant57/1 -> Bus Creator/73  "RVY2"
  Constant58/1 -> Bus Creator/74  "RVY3"
  Constant59/1 -> Bus Creator/75  "RVY4"
  Constant60/1 -> Bus Creator/76  "RVY5"
  Constant61/1 -> Bus Creator/77  "RVY6"
  Constant62/1 -> Bus Creator/78  "PTY1"
  Constant63/1 -> Bus Creator/79  "PTY2"
  Constant64/1 -> Bus Creator/80  "QSY1"
  Constant65/1 -> Bus Creator/81  "QSY2"
  Constant66/1 -> Bus Creator/82  "QSY3"
  Constant67/1 -> Bus Creator/83  "QSY4"
  Constant68/1 -> Bus Creator/84  "QBZ1"
  Constant69/1 -> Bus Creator/85  "QBZ2"
  Constant70/1 -> Bus Creator/86  "QBZ3"
  Constant71/1 -> Bus Creator/87  "QBZ4"
  Constant72/1 -> Bus Creator/88  "QBZ5"
  Constant73/1 -> Bus Creator/89  "QBZ9"
  Constant74/1 -> Bus Creator/90  "QBZ10"
  Constant75/1 -> Bus Creator/91  "QCZ1"
  Constant76/1 -> Bus Creator/92  "QDZ1"
  Constant77/1 -> Bus Creator/93  "QDZ2"
  Constant78/1 -> Bus Creator/94  "QDZ3"
  Constant79/1 -> Bus Creator/95  "QDZ4"
  Constant80/1 -> Bus Creator/96  "QDZ6"
  Constant110/1 -> Bus Creator/97  "QDZ7"
  Constant111/1 -> Bus Creator/98  "QDZ8"
  Constant112/1 -> Bus Creator/99  "QDZ9"
  Constant113/1 -> Bus Creator/100  "QEZ1"
  Constant114/1 -> Bus Creator/101  "QEZ2"
  Constant115/1 -> Bus Creator/102  "QEZ3"
  Constant122/1 -> Bus Creator/103  "QEZ4"
  Constant123/1 -> Bus Creator/104  "QEZ5"
  Constant124/1 -> Bus Creator/105  "QHZ1"
  Constant125/1 -> Bus Creator/106  "QHZ2"
  Constant126/1 -> Bus Creator/107  "QHZ3"
  Constant127/1 -> Bus Creator/108  "QHZ4"
  Constant116/1 -> Bus Creator/109  "SSZ1"
  Constant117/1 -> Bus Creator/110  "SSZ2"
  Constant118/1 -> Bus Creator/111  "SSZ3"
  Constant119/1 -> Bus Creator/112  "SSZ4"
  Constant120/1 -> Bus Creator/113  "QTZ1"
  Constant121/1 -> Bus Creator/114  "MBELT"
  Constant81/1 -> Bus Creator/4  "VERTICAL_STIFFNESS"
  Constant130/1 -> Bus Creator/8  "FZMIN"
  Constant131/1 -> Bus Creator/12  "KPUMIN"
  Constant132/1 -> Bus Creator/13  "KPUMAX"
  Constant133/1 -> Bus Creator/14  "ALPMIN"
  Constant134/1 -> Bus Creator/15  "ALPMAX"
  Constant135/1 -> Bus Creator/3  "TYRESIDE"
  Constant136/1 -> Bus Creator/17  "VERTICAL_DAMPING"
  Constant171/1 -> Bus Creator2/7  "FREFF"
  Constant170/1 -> Bus Creator2/6  "DREFF"
  Constant273/1 -> Bus Creator2/5  "BREFF"
  Constant138/1 -> Bus Creator3/1  "LFZO"
  Constant186/1 -> Bus Creator3/2  "LCX"
  Constant197/1 -> Bus Creator3/3  "LMUX"
  Constant208/1 -> Bus Creator3/4  "LEX"
  Constant219/1 -> Bus Creator3/5  "LKX"
  Constant230/1 -> Bus Creator3/6  "LHX"
  Constant241/1 -> Bus Creator3/7  "LVX"
  Constant195/1 -> Bus Creator3/8  "LGAX"
  Constant252/1 -> Bus Creator3/9  "LCY"
  Constant263/1 -> Bus Creator3/10  "LMUY"
  Constant139/1 -> Bus Creator3/11  "LEY"
  Constant150/1 -> Bus Creator3/12  "LKY"
  Constant161/1 -> Bus Creator3/13  "LHY"
  Constant172/1 -> Bus Creator3/14  "LVY"
  Constant180/1 -> Bus Creator3/15  "LGAY"
  Constant181/1 -> Bus Creator3/16  "LTR"
  Constant182/1 -> Bus Creator3/17  "LRES"
  Constant183/1 -> Bus Creator3/18  "LGAZ"
  Constant184/1 -> Bus Creator3/19  "LXAL"
  Constant185/1 -> Bus Creator3/20  "LYKA"
  Constant187/1 -> Bus Creator3/21  "LVYKA"
  Constant188/1 -> Bus Creator3/22  "LS"
  Constant189/1 -> Bus Creator3/23  "LSGKP"
  Constant190/1 -> Bus Creator3/24  "LSGAL"
  Constant191/1 -> Bus Creator3/25  "LGYR"
  Constant192/1 -> Bus Creator3/26  "LMX"
  Constant193/1 -> Bus Creator3/27  "LVMX"
  Constant194/1 -> Bus Creator3/28  "LMY"
  Constant137/1 -> Bus Creator2/1  "UNLOADED_RADIUS"
  Constant198/1 -> Bus Creator2/2  "FNOMIN"
  Constant255/1 -> Bus Creator2/19  "PCX1"
  Constant256/1 -> Bus Creator2/20  "PDX1"
  Constant257/1 -> Bus Creator2/21  "PDX2"
  Constant258/1 -> Bus Creator2/22  "PDX3"
  Constant259/1 -> Bus Creator2/23  "PEX1"
  Constant260/1 -> Bus Creator2/24  "PEX2"
  Constant261/1 -> Bus Creator2/25  "PEX3"
  Constant262/1 -> Bus Creator2/26  "PEX4"
  Constant264/1 -> Bus Creator2/27  "PKX1"
  Constant265/1 -> Bus Creator2/28  "PKX2"
  Constant266/1 -> Bus Creator2/29  "PKX3"
  Constant267/1 -> Bus Creator2/30  "PHX1"
  Constant268/1 -> Bus Creator2/31  "PHX2"
  Constant269/1 -> Bus Creator2/32  "PVX1"
  Constant270/1 -> Bus Creator2/33  "PVX2"
  Constant271/1 -> Bus Creator2/34  "RBX1"
  Constant272/1 -> Bus Creator2/35  "RBX2"
  Constant140/1 -> Bus Creator2/36  "RCX1"
  Constant141/1 -> Bus Creator2/37  "REX1"
  Constant142/1 -> Bus Creator2/38  "REX2"
  Constant143/1 -> Bus Creator2/39  "RHX1"
  Constant144/1 -> Bus Creator2/40  "PTX1"
  Constant145/1 -> Bus Creator2/41  "PTX2"
  Constant146/1 -> Bus Creator2/42  "PTX3"
  Constant147/1 -> Bus Creator2/43  "QSX1"
  Constant148/1 -> Bus Creator2/44  "QSX2"
  Constant149/1 -> Bus Creator2/45  "QSX3"
  Constant196/1 -> Bus Creator2/46  "PCY1"
  Constant199/1 -> Bus Creator2/47  "PDY1"
  Constant200/1 -> Bus Creator2/48  "PDY2"
  Constant201/1 -> Bus Creator2/49  "PDY3"
  Constant202/1 -> Bus Creator2/50  "PEY1"
  Constant203/1 -> Bus Creator2/51  "PEY2"
  Constant204/1 -> Bus Creator2/52  "PEY3"
  Constant205/1 -> Bus Creator2/53  "PEY4"
  Constant206/1 -> Bus Creator2/54  "PKY1"
  Constant207/1 -> Bus Creator2/55  "PKY2"
  Constant209/1 -> Bus Creator2/56  "PKY3"
  Constant210/1 -> Bus Creator2/57  "PHY1"
  Constant211/1 -> Bus Creator2/58  "PHY2"
  Constant212/1 -> Bus Creator2/59  "PHY3"
  Constant213/1 -> Bus Creator2/60  "PVY1"
  Constant214/1 -> Bus Creator2/61  "PVY2"
  Constant215/1 -> Bus Creator2/62  "PVY3"
  Constant216/1 -> Bus Creator2/63  "PVY4"
  Constant217/1 -> Bus Creator2/64  "RBY1"
  Constant218/1 -> Bus Creator2/65  "RBY2"
  Constant220/1 -> Bus Creator2/66  "RBY3"
  Constant221/1 -> Bus Creator2/67  "RCY1"
  Constant222/1 -> Bus Creator2/68  "REY1"
  Constant223/1 -> Bus Creator2/69  "REY2"
  Constant224/1 -> Bus Creator2/70  "RHY1"
  Constant225/1 -> Bus Creator2/71  "RHY2"
  Constant226/1 -> Bus Creator2/72  "RVY1"
  Constant227/1 -> Bus Creator2/73  "RVY2"
  Constant228/1 -> Bus Creator2/74  "RVY3"
  Constant229/1 -> Bus Creator2/75  "RVY4"
  Constant231/1 -> Bus Creator2/76  "RVY5"
  Constant232/1 -> Bus Creator2/77  "RVY6"
  Constant233/1 -> Bus Creator2/78  "PTY1"
  Constant234/1 -> Bus Creator2/79  "PTY2"
  Constant235/1 -> Bus Creator2/80  "QSY1"
  Constant236/1 -> Bus Creator2/81  "QSY2"
  Constant237/1 -> Bus Creator2/82  "QSY3"
  Constant238/1 -> Bus Creator2/83  "QSY4"
  Constant239/1 -> Bus Creator2/84  "QBZ1"
  Constant240/1 -> Bus Creator2/85  "QBZ2"
  Constant242/1 -> Bus Creator2/86  "QBZ3"
  Constant243/1 -> Bus Creator2/87  "QBZ4"
  Constant244/1 -> Bus Creator2/88  "QBZ5"
  Constant245/1 -> Bus Creator2/89  "QBZ9"
  Constant246/1 -> Bus Creator2/90  "QBZ10"
  Constant247/1 -> Bus Creator2/91  "QCZ1"
  Constant248/1 -> Bus Creator2/92  "QDZ1"
  Constant249/1 -> Bus Creator2/93  "QDZ2"
  Constant250/1 -> Bus Creator2/94  "QDZ3"
  Constant251/1 -> Bus Creator2/95  "QDZ4"
  Constant253/1 -> Bus Creator2/96  "QDZ6"
  Constant151/1 -> Bus Creator2/97  "QDZ7"
  Constant152/1 -> Bus Creator2/98  "QDZ8"
  Constant153/1 -> Bus Creator2/99  "QDZ9"
  Constant154/1 -> Bus Creator2/100  "QEZ1"
  Constant155/1 -> Bus Creator2/101  "QEZ2"
  Constant156/1 -> Bus Creator2/102  "QEZ3"
  Constant164/1 -> Bus Creator2/103  "QEZ4"
  Constant165/1 -> Bus Creator2/104  "QEZ5"
  Constant166/1 -> Bus Creator2/105  "QHZ1"
  Constant167/1 -> Bus Creator2/106  "QHZ2"
  Constant168/1 -> Bus Creator2/107  "QHZ3"
  Constant169/1 -> Bus Creator2/108  "QHZ4"
  Constant157/1 -> Bus Creator2/109  "SSZ1"
  Constant158/1 -> Bus Creator2/110  "SSZ2"
  Constant159/1 -> Bus Creator2/111  "SSZ3"
  Constant160/1 -> Bus Creator2/112  "SSZ4"
  Constant162/1 -> Bus Creator2/113  "QTZ1"
  Constant163/1 -> Bus Creator2/114  "MBELT"
  Constant254/1 -> Bus Creator2/4  "VERTICAL_STIFFNESS"
  Constant173/1 -> Bus Creator2/8  "FZMIN"
  Constant174/1 -> Bus Creator2/12  "KPUMIN"
  Constant175/1 -> Bus Creator2/13  "KPUMAX"
  Constant176/1 -> Bus Creator2/14  "ALPMIN"
  Constant177/1 -> Bus Creator2/15  "ALPMAX"
  Constant178/1 -> Bus Creator2/3  "TYRESIDE"
  Constant179/1 -> Bus Creator2/17  "VERTICAL_DAMPING"
  Constant274/1 -> Bus Creator2/115  "PIO"
  Constant275/1 -> Bus Creator2/116  "PPX1"
  Constant276/1 -> Bus Creator2/117  "PPX2"
  Constant277/1 -> Bus Creator2/118  "PPX3"
  Constant278/1 -> Bus Creator2/119  "PPX4"
  Constant279/1 -> Bus Creator2/120  "PPY1"
  Constant280/1 -> Bus Creator2/121  "PPY2"
  Constant281/1 -> Bus Creator2/122  "PPY3"
  Constant282/1 -> Bus Creator2/123  "PPY4"
  Constant283/1 -> Bus Creator2/124  "QPZ1"
  Constant284/1 -> Bus Creator/115  "PIO"
  Constant285/1 -> Bus Creator/116  "PPX1"
  Constant286/1 -> Bus Creator/117  "PPX2"
  Constant287/1 -> Bus Creator/118  "PPX3"
  Constant288/1 -> Bus Creator/119  "PPX4"
  Constant289/1 -> Bus Creator/120  "PPY1"
  Constant290/1 -> Bus Creator/121  "PPY2"
  Constant291/1 -> Bus Creator/122  "PPY3"
  Constant292/1 -> Bus Creator/123  "PPY4"
  Constant293/1 -> Bus Creator/124  "QPZ1"
  Constant294/1 -> Bus Creator2/9  "FZMAX"
  Constant296/1 -> Bus Creator2/11  "CAMMAX"
  Constant295/1 -> Bus Creator2/10  "CAMMIN"
  Constant297/1 -> Bus Creator2/16  "LONGVL"
  Constant298/1 -> Bus Creator/9  "FZMAX"
  Constant299/1 -> Bus Creator/10  "CAMMIN"
  Constant300/1 -> Bus Creator/11  "CAMMAX"
  Constant301/1 -> Bus Creator/16  "LONGVL"
  Constant302/1 -> Bus Creator2/18  "LOADINDEX"
  Constant303/1 -> Bus Creator/18  "LOADINDEX"

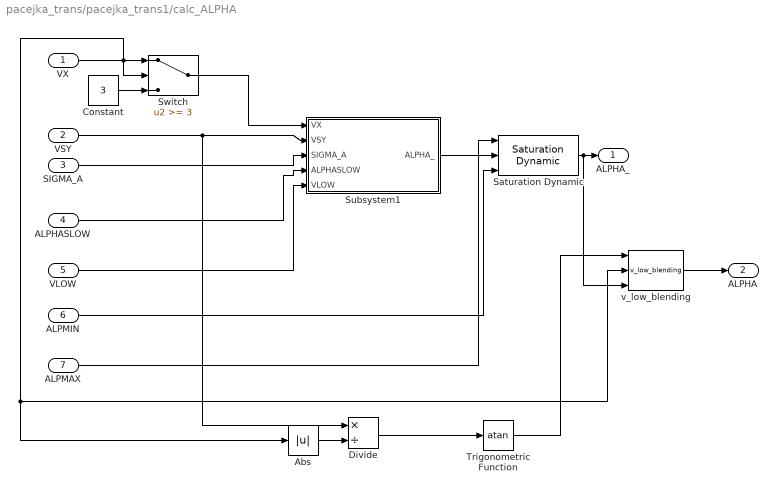
== system pacejka_trans/pacejka_trans1/calc_ALPHA ==
  VX : Inport
  VSY : Inport  Port=2
  SIGMA_A : Inport  Port=3
  ALPHASLOW : Inport  Port=4
  VLOW : Inport  Port=5
  ALPMIN : Inport  Port=6
  ALPMAX : Inport  Port=7
  Abs : Abs
  Constant : Constant  Value=3  VectorParams1D=off
  Divide : Product  Inputs=*/
  Saturation Dynamic : simulink/Discontinuities/Saturation Dynamic  OutMin=[]  OutMax=[]  OutDataTypeStr=Inherit: Same as second input  OutDataType=fixdt(1, 16)  OutScaling=2^-10  DoSatur=off
  Subsystem1 : Subsystem
  Switch : Switch  Threshold=3
  Trigonometric Function : Trigonometry  Operator=atan
  "v_low_blending " : $bdroot/pacejka_trans1/calc_KAPPA_/v_low_blending   SystemSampleTime=-1
  ALPHA_ : Outport  VectorParamsAs1DForOutWhenUnconnected=off
  ALPHA : Outport  Port=2  VectorParamsAs1DForOutWhenUnconnected=off
  wires:
  ALPHASLOW/1 -> Subsystem1/4(ALPHASLOW)
  VLOW/1 -> Subsystem1/5(VLOW)
  VSY/1 -> Divide/1, Subsystem1/2(VSY)
  Subsystem1/1(ALPHA_) -> Saturation Dynamic/2
  SIGMA_A/1 -> Subsystem1/3(SIGMA_A)
  VX/1 -> Abs/1, "v_low_blending "/2, Switch/1, Switch/2
  Switch/1 -> Subsystem1/1(VX)
  Constant/1 -> Switch/3
  Saturation Dynamic/1 -> "v_low_blending "/3, ALPHA_/1
  ALPMIN/1 -> Saturation Dynamic/3
  ALPMAX/1 -> Saturation Dynamic/1
  Abs/1 -> Divide/2
  Divide/1 -> Trigonometric Function/1
  "v_low_blending "/1 -> ALPHA/1
  Trigonometric Function/1 -> "v_low_blending "/1

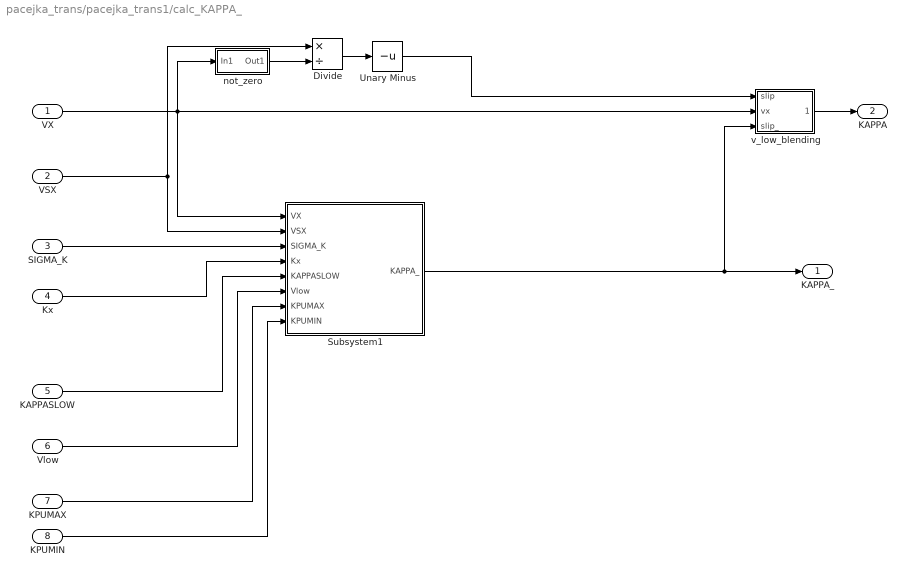
== system pacejka_trans/pacejka_trans1/calc_KAPPA_ ==
  VX : Inport
  VSX : Inport  Port=2
  SIGMA_K : Inport  Port=3
  Kx : Inport  Port=4
  KAPPASLOW : Inport  Port=5
  Vlow : Inport  Port=6
  KPUMAX : Inport  Port=7
  KPUMIN : Inport  Port=8
  Divide : Product  Inputs=*/
  Subsystem1 : Subsystem
  Unary Minus : UnaryMinus
  not_zero : Subsystem
  "v_low_blending " : Subsystem
  KAPPA_ : Outport  VectorParamsAs1DForOutWhenUnconnected=off
  KAPPA : Outport  Port=2  VectorParamsAs1DForOutWhenUnconnected=off
  wires:
  KPUMIN/1 -> Subsystem1/8(KPUMIN)
  KPUMAX/1 -> Subsystem1/7(KPUMAX)
  Vlow/1 -> Subsystem1/6(Vlow)
  KAPPASLOW/1 -> Subsystem1/5(KAPPASLOW)
  Kx/1 -> Subsystem1/4(Kx)
  SIGMA_K/1 -> Subsystem1/3(SIGMA_K)
  VSX/1 -> Divide/1, Subsystem1/2(VSX)
  VX/1 -> Subsystem1/1(VX), "v_low_blending "/2(vx), not_zero/1(In1)
  Divide/1 -> Unary Minus/1
  Subsystem1/1(KAPPA_) -> "v_low_blending "/3(slip_), KAPPA_/1
  Unary Minus/1 -> "v_low_blending "/1(slip)
  "v_low_blending "/1(slip_out) -> KAPPA/1
  not_zero/1(Out1) -> Divide/2
